simulink model "mech_car_handling"  (Simulink 7.1)
settings: Solver=ode15s  StartTime=0.0  StopTime=150  RelTol=1e-3
PostLoadFcn:
  | %%%%%%%%%%%%%%%%%%%%%%%%%%%%%%%%%%%%%%%%%%%%%%%%%%%%%%%%%%%%%%%%%%%%%%%%%%%
  | % INITIALIZE VEHICLE PARAMETERS
  | %%%%%%%%%%%%%%%%%%%%%%%%%%%%%%%%%%%%%%%%%%%%%%%%%%%%%%%%%%%%%%%%%%%%%%%%%%%
  | %clear;
  | %echo on;
  | 
  | % INITIALIZE STRUCTURES
  | chassis = struct();
  | wheel = struct();
  | axle = struct();
  | 
  | % INITIALIZE CHASSIS PARAMETERS
  | chassis.a = 1.50;          % longitudinal distance from CG to front axle
  | chassis.b = 0.99;           % longitudinal distance from CG to rear axle
  | chassis.w = 0.9;           % chassis width (wheel to wheel distance)
  | chassis.hu = 0.1;          % height of unsprung mass above ground
  | chassis.hs = 0.3;          % height of sprung mass above unsprung mass
  | chassis.ms = 1470;      % mass of sprung mass
  | chassis.mu = 200;        % mass of unsprung mass
  | 
  | % INITIALIZE WHEEL PARAMETERS
  | wheel.r = 0.3;             % wheel radius
  | wheel.m = 30;            % wheel mass
  | wheel.I = [0.52 0 0;0 1 0;0 0 0.52];
  | 
  | % INITIALIZE AXLE PARAMETERS
  | axle.m = 2;                 % axle mass
  | 
  | % COMPUTE STEADY STATE LOADS
  | Fzf = 0.5*(chassis.ms+chassis.mu) * 9.81 * chassis.b / (chassis.a + chassis.b);    % initial front wheel reaction
  | Fzr = 0.5*(chassis.ms+chassis.mu) * 9.81 * chassis. a / (chassis.a + chassis.b);    % initial rear wheel reaction
  | 
  | % INITIALIZE ROLL PARAMETERS
  | kf = 9000;                 % sprung front roll stiffness
  | kb = 5500;                % sprung rear roll stiffness
  | ku = 10000;              % unsprung roll stiffness (same front and rear)
  | bu = 0.1 * ku;            % unsprung roll damping
  | kr = kf + kb;              % total sprung roll stiffness
  | br = 0.1*kr;                % sprung roll damping
  | 
  | % INITIALIZE NONLINEAR TIRE MODEL PARAMETERS
  | a1 = 1.8658e-5;            % nonlinear tire model proportional coefficient
  | a2 = 9.3290e-4;            % nonlinear tire model quadratic coefficient
  | 
  | % INITIALIZE CONTROLLER PARAMETERS
  | Kp = 10000;                 % speed controller proportional gain
  | 
  | % INITIALIZE STEERING PARAMETERS
  | steeringAngle = 2;
  | %echo off;
StopFcn:
  | appDataName = 'mech_car_steering_fig_data';
  | mech_car_handling_fig_mgr('init',appDataName);
  | 
  | p = size(speed.signals.values);
  | p = p(1);
  | R = speed.signals.values([30:p])./yaw_rate.signals.values([30:p]);
  | modelFigure = getappdata(0,'mech_car_steering_fig_data');
  | plot(speed.signals.values([30:p]),R,'g','Parent',modelFigure.axesH);
libraries: mblibv1 x33, simulink x3
(part 2 of 2)

== system mech_car_handling/Unsprung System/UNSPRUNG MASS ==
  Body : mblibv1/Bodies/Body  DialogController=MECH.DynMechDlgSource  PhysicalDomain=mechanical  SubClassName=Unknown  LeftPortType=workingframe  RightPortType=workingframe  LConnTagsString=CG  RConnTagsString=CS3  DialogClass=MechanicalBodyBlock  Mass=m  MassUnits=kg  InertiaUnits=kg*m^2  Inertia=eye(3)  Shape=Cylinder  ShapeDims=[1 1]  ShapeUnits=m  ShapeUse=false  Density=1  DensityUnits=kg/m^3  DensityUse=false  GraphicsMode=1  BodyColor=[0.5 0.5 0.5]  GraphicsObj=[]  AttachedToCS=1  CG=Left$CG$[0 0 h]$CS3$CS3$m$[0 0 0]$Euler X-Y-Z$deg$WORLD$true  WorkingFrames=Right$CS1$[0 0 0]$CG$CG$m$[0 0 0]$Euler X-Y-Z$deg$WORLD$false#Right$CS3$[0 0 0]$ADJOINING$ADJOINING$m$[0 0 0]$Euler X-Y-Z$deg$WORLD$true  CGPos=[0 0 h]  CGRot=[0 0 0]  CS0Pos=[]  CS0Rot=[]  CS1Pos=[0 0 0]  CS1Rot=[0 0 0]  CS2Pos=[]  CS2Rot=[]  CS3Pos=[0 0 0]  CS3Rot=[0 0 0]  CS4Pos=[]  CS4Rot=[]  CS5Pos=[]  CS5Rot=[]  CS6Pos=[]  CS6Rot=[]  CS7Pos=[]  CS7Rot=[]  CS8Pos=[]  CS8Rot=[]  CS9Pos=[]  CS9Rot=[]  CS10Pos=[]  CS10Rot=[]  CS11Pos=[]  CS11Rot=[]  CS12Pos=[]  CS12Rot=[]  CS13Pos=[]  CS13Rot=[]  CS14Pos=[]  CS14Rot=[]  CS15Pos=[]  CS15Rot=[]  CS16Pos=[]  CS16Rot=[]  CS17Pos=[]  CS17Rot=[]  CS18Pos=[]  CS18Rot=[]  CS19Pos=[]  CS19Rot=[]  CS20Pos=[]  CS20Rot=[]
  TO AXLES : PMIOPort  Orientation=left  Port=1  Side=Right
  TO M SPRUNG : PMIOPort  Port=2  Side=Left
  connections:
  Body/RConn1 -- TO AXLES/RConn1
  TO M SPRUNG/RConn1 -- Body/LConn1
